simulink model "dds_test"  (Simulink 7.4)
settings: Solver=ode45  StartTime=0.0  StopTime=1000  RelTol=1e-3
libraries: xbsIndex_r4 x23, simulink x2
(part 1 of 5)
settings Model: Creator=chenhong  LastModifiedBy=chenhong

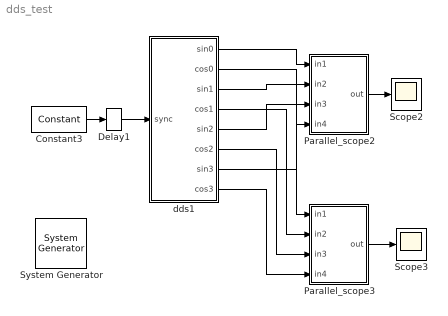
== system dds_test ==
  " System Generator" : xbsIndex_r4/ System Generator  Tag=genX  SystemSampleTime=-1  xilinxfamily=Virtex6  part=xc6vsx315t  speed=-3  package=ff1156  synthesis_tool=XST  clock_wrapper=Clock Enables  directory=./netlist  testbench=off  simulink_period=1  sysclk_period=10  dcm_input_clock_period=10  incr_netlist=off  trim_vbits=Everywhere in SubSystem  dbl_ovrd=According to Block Masks  core_generation=According to Block Masks  run_coregen=off  deprecated_control=off  eval_field=0  block_type=sysgen
      settings: block_version=11.4
  Constant3 : xbsIndex_r4/Constant  arith_type=Boolean  const=1  n_bits=16  bin_pt=14  explicit_period=on  period=1024  equ=P=C  opselect=C  inp2=PCIN>>17  opr=+  inp1=P  carry=CIN  dbl_ovrd=off  block_type=constant
      settings: block_version=11.4
  Delay1 : xbsIndex_r4/Delay  en=off  latency=25  dbl_ovrd=off  reg_retiming=off  block_type=delay
      settings: block_version=11.4
  Parallel_scope2 : Subsystem  AncestorBlock=xblocks_library_scopes/Parallel_scope  mask(Parallel Scope){n_inputs=4, sample_period=1}
      mask prompts: n_inputs "Number of inputs"; sample_period "Sample Period"
      mask help:
      | This parallel scope can handle parallel inputs
      | by propagating though gateways and serialize into
      | one single stream. The output can then be connected
      | directly to a scope or toWorkspace.
      |
      | The sample_period desribes the parallel inputs rate.
      | For example, for a 4-inputs stream with sample_period = 1
      | (4 parallel inputs per Clk),  the output stream frequency
      | would be 4/1 = 4 (Sample/Clk)
      mask init:
      | config.source=str2func('parallel_scope_init_xblock');
      | config.depend=get_dependlist('parallel_scope');
      | config.toplevel=gcb;
      | set_param(gcb,'LinkStatus','inactive');
      | xBlock(config, {config.toplevel,...
      |     'n_inputs', n_inputs, ...
      |     'sample_period', sample_period});
      settings: AttributesFormatString=Sample Period = 1
  Parallel_scope3 : Subsystem  AncestorBlock=xblocks_library_scopes/Parallel_scope  mask(Parallel Scope){n_inputs=4, sample_period=1}
      mask prompts: n_inputs "Number of inputs"; sample_period "Sample Period"
      mask help:
      | This parallel scope can handle parallel inputs
      | by propagating though gateways and serialize into
      | one single stream. The output can then be connected
      | directly to a scope or toWorkspace.
      |
      | The sample_period desribes the parallel inputs rate.
      | For example, for a 4-inputs stream with sample_period = 1
      | (4 parallel inputs per Clk),  the output stream frequency
      | would be 4/1 = 4 (Sample/Clk)
      mask init: same as dds_test/Parallel_scope2
      settings: AttributesFormatString=Sample Period = 1
  Scope2 : Scope
  Scope3 : Scope
  dds1 : Subsystem  AncestorBlock=xblocks_library_downconverter/dds  mask(dds){freq_div=2048, freq=1, num_lo=4, n_bits=8, latency=2}
      mask prompts: freq_div "Frequency divisions (M)"; freq "Frequency (? / M*2pi)"; num_lo "Parallel LOs"; n_bits "Bit Width"
      mask help:
      | Generates P channels of sin and cos data for mixing
      | with input data in a DDC. To generate frequency
      | N/M(Fc x P) (where Fc is the clock rate)
      | M = "Frequency Divisions", N = "Frequency",
      | Parallel LOs = P
      mask init:
      | config.source=str2func('dds_init_xblock');
      | config.depend=get_dependlist('dds');
      | config.toplevel=gcb;
      | set_param(gcb,'LinkStatus','inactive');
      | xBlock(config, {config.toplevel,...
      |     'freq_div', freq_div, ...
      |     'freq', freq, ...
      |     'num_lo', num_lo, ...
      |     'n_bits', n_bits, ...
      |     'latency', latency});
      settings: AttributesFormatString=lo at -1/2048
      mask Help: eval('xlWeb(''http://casper.berkeley.edu/wiki/Dds'')')
  wires:
  dds1/1(sin0) -> Parallel_scope2/1(in1)
  dds1/3(sin1) -> Parallel_scope2/2(in2)
  dds1/5(sin2) -> Parallel_scope2/3(in3)
  dds1/7(sin3) -> Parallel_scope2/4(in4)
  dds1/2(cos0) -> Parallel_scope3/1(in1)
  dds1/4(cos1) -> Parallel_scope3/2(in2)
  dds1/6(cos2) -> Parallel_scope3/3(in3)
  dds1/8(cos3) -> Parallel_scope3/4(in4)
  Parallel_scope2/1(out) -> Scope2/1
  Parallel_scope3/1(out) -> Scope3/1
  Constant3/1 -> Delay1/1
  Delay1/1 -> dds1/1(sync)

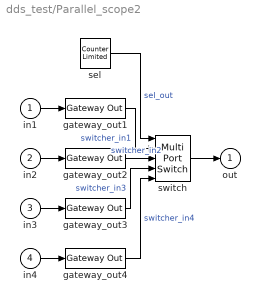
== system dds_test/Parallel_scope2 ==
  in1 : Inport
  in2 : Inport  Port=2
  in3 : Inport  Port=3
  in4 : Inport  Port=4
  gateway_out{1..4} (4 alike) : xbsIndex_r4/Gateway Out  hdl_port=off  timing_constraint=None  locs_specified=off  LOCs={}  block_type=gatewayout
      settings: infoedit="Gateway out block.  Converts Xilinx fixed point inputs into ouputs of type Simulink integer, double, or fixed point.<br><br>Hardware notes:  In hardware these blocks become top level output ports or are discarded, depending on how they are configured."  block_version=11.4
  sel : simulink/Sources/Counter Limited  SystemSampleTime=-1  uplimit=3  tsamp=0.25
  switch : MultiPortSwitch  Inputs=4  zeroidx=on  OutDataType=fixdt(1, 16)  OutScaling=2^0
  out : Outport
  wires:
  switch/1 -> out/1
  gateway_out4/1 -> switch/5  "switcher_in4"
  gateway_out3/1 -> switch/4  "switcher_in3"
  gateway_out2/1 -> switch/3  "switcher_in2"
  gateway_out1/1 -> switch/2  "switcher_in1"
  sel/1 -> switch/1  "sel_out"
  in4/1 -> gateway_out4/1
  in3/1 -> gateway_out3/1
  in2/1 -> gateway_out2/1
  in1/1 -> gateway_out1/1

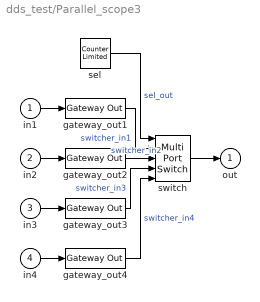
== system dds_test/Parallel_scope3 ==
  in1 : Inport
  in2 : Inport  Port=2
  in3 : Inport  Port=3
  in4 : Inport  Port=4
  gateway_out{1..4} (4 alike) : xbsIndex_r4/Gateway Out  hdl_port=off  timing_constraint=None  locs_specified=off  LOCs={}  block_type=gatewayout
      settings: infoedit="Gateway out block.  Converts Xilinx fixed point inputs into ouputs of type Simulink integer, double, or fixed point.<br><br>Hardware notes:  In hardware these blocks become top level output ports or are discarded, depending on how they are configured."  block_version=11.4
  sel : simulink/Sources/Counter Limited  SystemSampleTime=-1  uplimit=3  tsamp=0.25
  switch : MultiPortSwitch  Inputs=4  zeroidx=on  OutDataType=fixdt(1, 16)  OutScaling=2^0
  out : Outport
  wires:
  switch/1 -> out/1
  gateway_out4/1 -> switch/5  "switcher_in4"
  gateway_out3/1 -> switch/4  "switcher_in3"
  gateway_out2/1 -> switch/3  "switcher_in2"
  gateway_out1/1 -> switch/2  "switcher_in1"
  sel/1 -> switch/1  "sel_out"
  in4/1 -> gateway_out4/1
  in3/1 -> gateway_out3/1
  in2/1 -> gateway_out2/1
  in1/1 -> gateway_out1/1

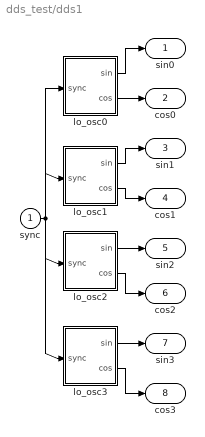
== system dds_test/dds1 ==
  sync : Inport
  lo_osc0 : Subsystem
  lo_osc1 : Subsystem
  lo_osc2 : Subsystem
  lo_osc3 : Subsystem
  sin0 : Outport  OutDataType=sfix(16)  OutScaling=2^0
  cos0 : Outport  Port=2  OutDataType=sfix(16)  OutScaling=2^0
  sin1 : Outport  Port=3  OutDataType=sfix(16)  OutScaling=2^0
  cos1 : Outport  Port=4  OutDataType=sfix(16)  OutScaling=2^0
  sin2 : Outport  Port=5  OutDataType=sfix(16)  OutScaling=2^0
  cos2 : Outport  Port=6  OutDataType=sfix(16)  OutScaling=2^0
  sin3 : Outport  Port=7  OutDataType=sfix(16)  OutScaling=2^0
  cos3 : Outport  Port=8  OutDataType=sfix(16)  OutScaling=2^0
  wires:
  sync/1 -> lo_osc3/1(sync), lo_osc2/1(sync), lo_osc1/1(sync), lo_osc0/1(sync)
  lo_osc3/2(cos) -> cos3/1
  lo_osc3/1(sin) -> sin3/1
  lo_osc2/2(cos) -> cos2/1
  lo_osc2/1(sin) -> sin2/1
  lo_osc1/2(cos) -> cos1/1
  lo_osc1/1(sin) -> sin1/1
  lo_osc0/2(cos) -> cos0/1
  lo_osc0/1(sin) -> sin0/1

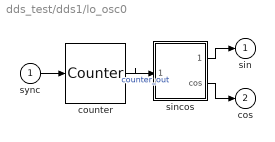
== system dds_test/dds1/lo_osc0 ==
  sync : Inport
  counter : xbsIndex_r4/Counter  cnt_type=Free Running  cnt_to=Inf  operation=Up  start_count=0  cnt_by_val=4  arith_type=Unsigned  n_bits=11  bin_pt=0  load_pin=off  rst=on  en=off  explicit_period=on  period=1  dbl_ovrd=off  use_behavioral_HDL=off  implementation=Fabric  block_type=counter
      settings: block_version=11.4
  sincos : Subsystem
      settings: AttributesFormatString=|
      | depth_bits = 11
      | bit_width = 8
  sin : Outport
  cos : Outport  Port=2
  wires:
  sincos/2(cos) -> cos/1
  sincos/1(-sine) -> sin/1
  counter/1 -> sincos/1(theta)  "counter_out"
  sync/1 -> counter/1

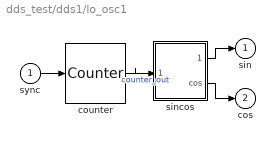
== system dds_test/dds1/lo_osc1 ==
  sync : Inport
  counter : xbsIndex_r4/Counter  cnt_type=Free Running  cnt_to=Inf  operation=Up  start_count=1  cnt_by_val=4  arith_type=Unsigned  n_bits=11  bin_pt=0  load_pin=off  rst=on  en=off  explicit_period=on  period=1  dbl_ovrd=off  use_behavioral_HDL=off  implementation=Fabric  block_type=counter
      settings: block_version=11.4
  sincos : Subsystem
      settings: AttributesFormatString=|
      | depth_bits = 11
      | bit_width = 8
  sin : Outport
  cos : Outport  Port=2
  wires:
  sincos/2(cos) -> cos/1
  sincos/1(-sine) -> sin/1
  counter/1 -> sincos/1(theta)  "counter_out"
  sync/1 -> counter/1

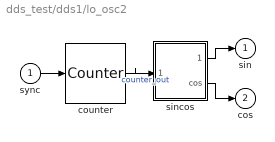
== system dds_test/dds1/lo_osc2 ==
  sync : Inport
  counter : xbsIndex_r4/Counter  cnt_type=Free Running  cnt_to=Inf  operation=Up  start_count=2  cnt_by_val=4  arith_type=Unsigned  n_bits=11  bin_pt=0  load_pin=off  rst=on  en=off  explicit_period=on  period=1  dbl_ovrd=off  use_behavioral_HDL=off  implementation=Fabric  block_type=counter
      settings: block_version=11.4
  sincos : Subsystem
      settings: AttributesFormatString=|
      | depth_bits = 11
      | bit_width = 8
  sin : Outport
  cos : Outport  Port=2
  wires:
  sincos/2(cos) -> cos/1
  sincos/1(-sine) -> sin/1
  counter/1 -> sincos/1(theta)  "counter_out"
  sync/1 -> counter/1

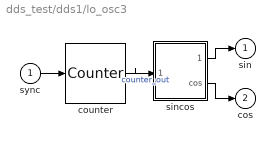
== system dds_test/dds1/lo_osc3 ==
  sync : Inport
  counter : xbsIndex_r4/Counter  cnt_type=Free Running  cnt_to=Inf  operation=Up  start_count=3  cnt_by_val=4  arith_type=Unsigned  n_bits=11  bin_pt=0  load_pin=off  rst=on  en=off  explicit_period=on  period=1  dbl_ovrd=off  use_behavioral_HDL=off  implementation=Fabric  block_type=counter
      settings: block_version=11.4
  sincos : Subsystem
      settings: AttributesFormatString=|
      | depth_bits = 11
      | bit_width = 8
  sin : Outport
  cos : Outport  Port=2
  wires:
  sincos/2(cos) -> cos/1
  sincos/1(-sine) -> sin/1
  counter/1 -> sincos/1(theta)  "counter_out"
  sync/1 -> counter/1
